simulink model "TurnLightLogic_backup"  (R2023a)
settings: Solver=FixedStepDiscrete  StartTime=0.0  StopTime=10.0  FixedStep=0.01  RelTol=1e-3
undefined symbols (not defined in the file or in its folder): ComplexTurnLightOnOff, ComplexTurnLightPosition, TurnLightCtrlPara, TurnLightService_TurnLightControl_Operation_Operation
settings Model: Creator=19856  LastModifiedBy=19856
settings DataIOCC: SaveFormat=StructureWithTime
settings OptimizationCC: DefaultParameterBehavior=Inlined  EnhancedBackFolding=on  PassReuseOutputArgsAs=Individual arguments  ZeroExternalMemoryAtStartup=off  ZeroInternalMemoryAtStartup=off  OptimizeBlockOrder=speed  DifferentSizesBufferReuse=on  OptimizationCustomize=off  EfficientTunableParamExpr=on
settings DebuggingCC: ParameterTunabilityLossMsg=error
settings ModelReferenceCC: ModelReferenceNumInstancesAllowed=Single
settings SFSimCC: MATLABDynamicMemAlloc=off
settings RTWCC: Description=AUTOSAR  SystemTargetFile=autosar.tlc  GenCodeOnly=on  TemplateMakefile=ert_default_tmf
settings CodeAppCC: ForceParamTrailComments=on  IgnoreCustomStorageClasses=off  OperatorAnnotations=on  SimulinkDataObjDesc=on  SFDataObjDesc=on  InsertBlockDesc=on
settings STFCustomTargetCC: MultiwordLength=256  ParMdlRefBuildCompliant=on  CompOptLevelCompliant=on  ConcurrentExecutionCompliant=off  IncludeMdlTerminateFcn=off  CombineOutputUpdateFcns=on  SuppressErrorStatus=on  ERTCustomFileBanners=on  SupportNonFinite=off  SupportComplex=off  SupportContinuousTime=off  SupportNonInlinedSFcns=off  RemoveResetFunc=on  MATLABClassNameForMDSCustomization=Simulink.SoftwareTarget.ERTCustomization  AutosarCompliant=on  GRTInterface=off  LookupTableObjectStructAxisOrder=2,1,3,4,...  LUTObjectStructOrderEvenSpacing=Size,Table,Breakpoints  SystemTargetFile=autosar.tlc
settings ERTTargetCC: TargetLangStandard=C99 (ISO)  ConcurrentExecutionCompliant=off  IncludeMdlTerminateFcn=off  SuppressErrorStatus=on  SupportNonFinite=off  SupportComplex=off  ModelStepFunctionPrototypeControlCompliant=off  CPPClassGenCompliant=off  AutosarCompliant=on  LookupTableObjectStructAxisOrder=2,1,3,4,...  LUTObjectStructOrderEvenSpacing=Size,Table,Breakpoints  InlinedParameterPlacement=NonHierarchical  ERTCustomFileTemplate=example_file_process.tlc

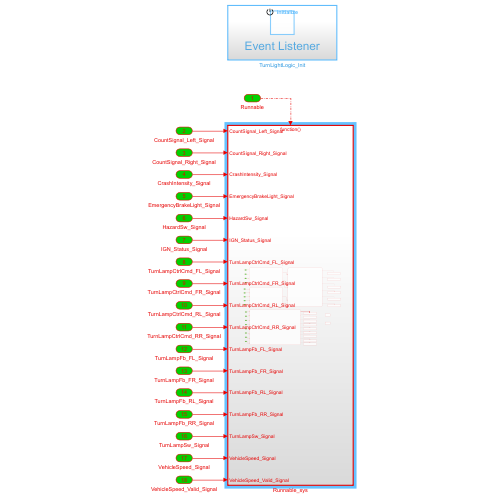
[thumbnail: Simulink's stored preview of the top-level diagram]
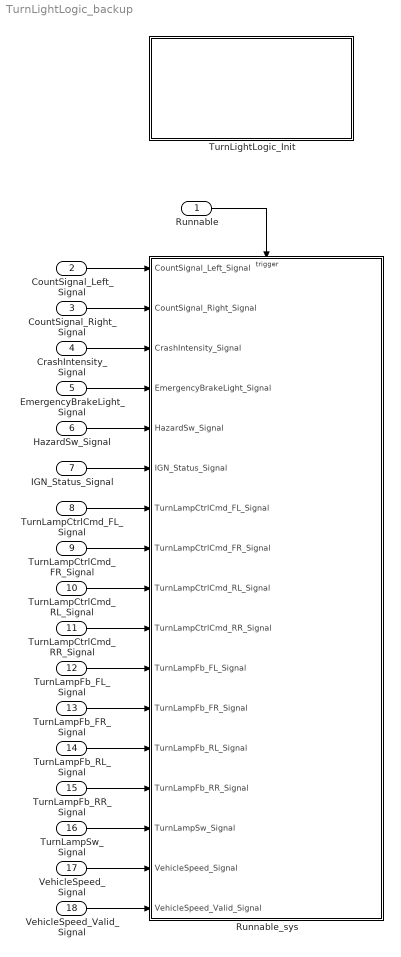
== system TurnLightLogic_backup ==
  Runnable : Inport  SampleTime=0.01  OutputFunctionCall=on
  CountSignal_Left_Signal : Inport  Port=2  OutDataTypeStr=uint8  PortDimensions=1
  CountSignal_Right_Signal : Inport  Port=3  OutDataTypeStr=uint8  PortDimensions=1
  CrashIntensity_Signal : Inport  Port=4  OutDataTypeStr=uint8  PortDimensions=1
  EmergencyBrakeLight_Signal : Inport  Port=5  OutDataTypeStr=uint8  PortDimensions=1
  HazardSw_Signal : Inport  Port=6  OutDataTypeStr=uint8  PortDimensions=1
  IGN_Status_Signal : Inport  Port=7  OutDataTypeStr=uint8  PortDimensions=1
  TurnLampCtrlCmd_FL_Signal : Inport  Port=8  OutDataTypeStr=uint8  PortDimensions=1
  TurnLampCtrlCmd_FR_Signal : Inport  Port=9  OutDataTypeStr=uint8  PortDimensions=1
  TurnLampCtrlCmd_RL_Signal : Inport  Port=10  OutDataTypeStr=uint8  PortDimensions=1
  TurnLampCtrlCmd_RR_Signal : Inport  Port=11  OutDataTypeStr=uint8  PortDimensions=1
  TurnLampFb_FL_Signal : Inport  Port=12  OutDataTypeStr=uint8  PortDimensions=1
  TurnLampFb_FR_Signal : Inport  Port=13  OutDataTypeStr=uint8  PortDimensions=1
  TurnLampFb_RL_Signal : Inport  Port=14  OutDataTypeStr=uint8  PortDimensions=1
  TurnLampFb_RR_Signal : Inport  Port=15  OutDataTypeStr=uint8  PortDimensions=1
  TurnLampSw_Signal : Inport  Port=16  OutDataTypeStr=uint8  PortDimensions=1
  VehicleSpeed_Signal : Inport  Port=17  OutDataTypeStr=uint8  PortDimensions=1
  VehicleSpeed_Valid_Signal : Inport  Port=18  OutDataTypeStr=uint8  PortDimensions=1
  Runnable_sys : Subsystem
  TurnLightLogic_Init : Subsystem
  wires:
  CountSignal_Left_Signal/1 -> Runnable_sys/1(CountSignal_Left_Signal)
  CountSignal_Right_Signal/1 -> Runnable_sys/2(CountSignal_Right_Signal)
  CrashIntensity_Signal/1 -> Runnable_sys/3(CrashIntensity_Signal)
  EmergencyBrakeLight_Signal/1 -> Runnable_sys/4(EmergencyBrakeLight_Signal)
  HazardSw_Signal/1 -> Runnable_sys/5(HazardSw_Signal)
  IGN_Status_Signal/1 -> Runnable_sys/6(IGN_Status_Signal)
  TurnLampCtrlCmd_FL_Signal/1 -> Runnable_sys/7(TurnLampCtrlCmd_FL_Signal)
  TurnLampCtrlCmd_FR_Signal/1 -> Runnable_sys/8(TurnLampCtrlCmd_FR_Signal)
  TurnLampCtrlCmd_RL_Signal/1 -> Runnable_sys/9(TurnLampCtrlCmd_RL_Signal)
  TurnLampCtrlCmd_RR_Signal/1 -> Runnable_sys/10(TurnLampCtrlCmd_RR_Signal)
  TurnLampFb_FL_Signal/1 -> Runnable_sys/11(TurnLampFb_FL_Signal)
  TurnLampFb_FR_Signal/1 -> Runnable_sys/12(TurnLampFb_FR_Signal)
  TurnLampFb_RL_Signal/1 -> Runnable_sys/13(TurnLampFb_RL_Signal)
  TurnLampFb_RR_Signal/1 -> Runnable_sys/14(TurnLampFb_RR_Signal)
  TurnLampSw_Signal/1 -> Runnable_sys/15(TurnLampSw_Signal)
  VehicleSpeed_Signal/1 -> Runnable_sys/16(VehicleSpeed_Signal)
  VehicleSpeed_Valid_Signal/1 -> Runnable_sys/17(VehicleSpeed_Valid_Signal)
  Runnable/1 -> Runnable_sys/Trigger

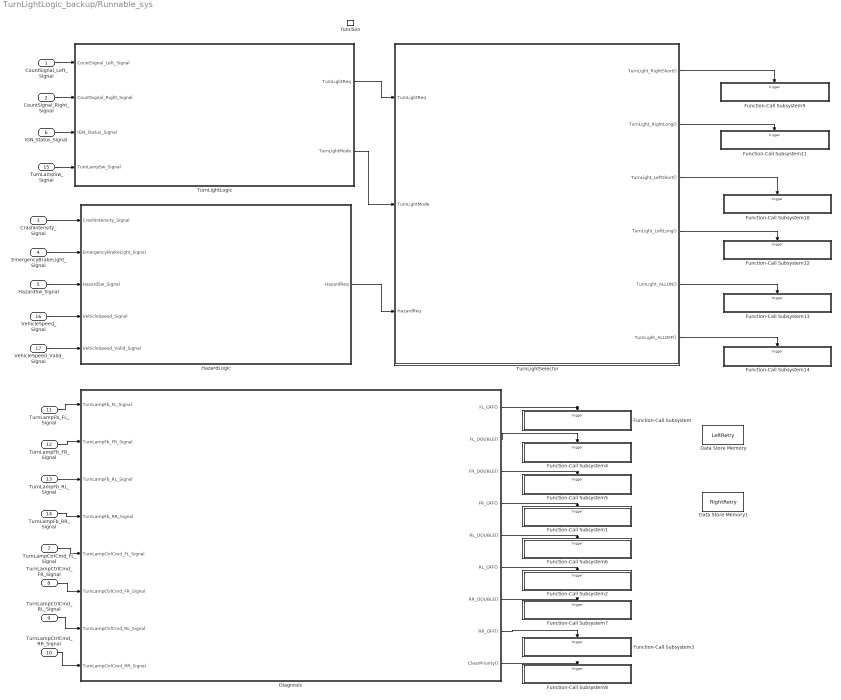
== system TurnLightLogic_backup/Runnable_sys ==
  CountSignal_Left_Signal : Inport
  CountSignal_Right_Signal : Inport  Port=2
  CrashIntensity_Signal : Inport  Port=3
  EmergencyBrakeLight_Signal : Inport  Port=4
  HazardSw_Signal : Inport  Port=5
  IGN_Status_Signal : Inport  Port=6
  TurnLampCtrlCmd_FL_Signal : Inport  Port=7
  TurnLampCtrlCmd_FR_Signal : Inport  Port=8
  TurnLampCtrlCmd_RL_Signal : Inport  Port=9
  TurnLampCtrlCmd_RR_Signal : Inport  Port=10
  TurnLampFb_FL_Signal : Inport  Port=11
  TurnLampFb_FR_Signal : Inport  Port=12
  TurnLampFb_RL_Signal : Inport  Port=13
  TurnLampFb_RR_Signal : Inport  Port=14
  TurnLampSw_Signal : Inport  Port=15
  VehicleSpeed_Signal : Inport  Port=16  OutDataTypeStr=uint8
  VehicleSpeed_Valid_Signal : Inport  Port=17
  function : TriggerPort  TriggerType=function-call  VariantControl=(inherit)  SampleTimeType=periodic  SampleTime=-1
  Data Store Memory : DataStoreMemory  DataStoreName=LeftRetry  WriteAfterWriteMsg=warning  ShowAdditionalParam=off  OutDataTypeStr=uint8
  Data Store Memory1 : DataStoreMemory  DataStoreName=RightRetry  WriteAfterWriteMsg=warning  ShowAdditionalParam=off  OutDataTypeStr=uint8
  Diagnosis : Stateflow chart  TreatAsAtomicUnit=on
  Function-Call Subsystem : Subsystem  TreatAsAtomicUnit=on
  Function-Call Subsystem1 : Subsystem  TreatAsAtomicUnit=on
  Function-Call Subsystem10 : Subsystem  TreatAsAtomicUnit=on
  Function-Call Subsystem11 : Subsystem  TreatAsAtomicUnit=on
  Function-Call Subsystem12 : Subsystem  TreatAsAtomicUnit=on
  Function-Call Subsystem13 : Subsystem  TreatAsAtomicUnit=on
  Function-Call Subsystem14 : Subsystem  TreatAsAtomicUnit=on
  Function-Call Subsystem2 : Subsystem  TreatAsAtomicUnit=on
  Function-Call Subsystem3 : Subsystem  TreatAsAtomicUnit=on
  Function-Call Subsystem4 : Subsystem  TreatAsAtomicUnit=on
  Function-Call Subsystem5 : Subsystem  TreatAsAtomicUnit=on
  Function-Call Subsystem6 : Subsystem  TreatAsAtomicUnit=on
  Function-Call Subsystem7 : Subsystem  TreatAsAtomicUnit=on
  Function-Call Subsystem8 : Subsystem  TreatAsAtomicUnit=on
  Function-Call Subsystem9 : Subsystem  TreatAsAtomicUnit=on
  HazardLogic : Stateflow chart  TreatAsAtomicUnit=on
  TurnLightLogic : Stateflow chart  TreatAsAtomicUnit=on
  TurnLightSelector : Stateflow chart  TreatAsAtomicUnit=on
  wires:
  CountSignal_Left_Signal/1 -> TurnLightLogic/1(CountSignal_Left_Signal)
  CountSignal_Right_Signal/1 -> TurnLightLogic/2(CountSignal_Right_Signal)
  CrashIntensity_Signal/1 -> HazardLogic/1(CrashIntensity_Signal)
  EmergencyBrakeLight_Signal/1 -> HazardLogic/2(EmergencyBrakeLight_Signal)
  HazardSw_Signal/1 -> HazardLogic/3(HazardSw_Signal)
  IGN_Status_Signal/1 -> TurnLightLogic/3(IGN_Status_Signal)
  TurnLampFb_FL_Signal/1 -> Diagnosis/1(TurnLampFb_FL_Signal)
  TurnLampFb_FR_Signal/1 -> Diagnosis/2(TurnLampFb_FR_Signal)
  TurnLampFb_RL_Signal/1 -> Diagnosis/3(TurnLampFb_RL_Signal)
  TurnLampFb_RR_Signal/1 -> Diagnosis/4(TurnLampFb_RR_Signal)
  TurnLampSw_Signal/1 -> TurnLightLogic/4(TurnLampSw_Signal)
  VehicleSpeed_Signal/1 -> HazardLogic/4(VehicleSpeed_Signal)
  VehicleSpeed_Valid_Signal/1 -> HazardLogic/5(VehicleSpeed_Valid_Signal)
  TurnLightLogic/1(TurnLightReq) -> TurnLightSelector/1(TurnLightReq)
  TurnLightLogic/2(TurnLightMode) -> TurnLightSelector/2(TurnLightMode)
  HazardLogic/1(HazardReq) -> TurnLightSelector/3(HazardReq)
  TurnLampCtrlCmd_FL_Signal/1 -> Diagnosis/5(TurnLampCtrlCmd_FL_Signal)
  TurnLampCtrlCmd_FR_Signal/1 -> Diagnosis/6(TurnLampCtrlCmd_FR_Signal)
  TurnLampCtrlCmd_RL_Signal/1 -> Diagnosis/7(TurnLampCtrlCmd_RL_Signal)
  TurnLampCtrlCmd_RR_Signal/1 -> Diagnosis/8(TurnLampCtrlCmd_RR_Signal)
  TurnLightSelector/6(TurnLight_ALLOFF()) -> Function-Call Subsystem14/Trigger
  TurnLightSelector/5(TurnLight_ALLON()) -> Function-Call Subsystem13/Trigger
  TurnLightSelector/4(TurnLight_LeftLong()) -> Function-Call Subsystem12/Trigger
  TurnLightSelector/3(TurnLight_LeftShort()) -> Function-Call Subsystem10/Trigger
  TurnLightSelector/2(TurnLight_RightLong()) -> Function-Call Subsystem11/Trigger
  TurnLightSelector/1(TurnLight_RightShort()) -> Function-Call Subsystem9/Trigger
  Diagnosis/1(FL_OFF()) -> Function-Call Subsystem/Trigger
  Diagnosis/2(FL_DOUBLE()) -> Function-Call Subsystem4/Trigger
  Diagnosis/3(FR_DOUBLE()) -> Function-Call Subsystem5/Trigger
  Diagnosis/4(FR_OFF()) -> Function-Call Subsystem1/Trigger
  Diagnosis/5(RL_DOUBLE()) -> Function-Call Subsystem6/Trigger
  Diagnosis/6(RL_OFF()) -> Function-Call Subsystem2/Trigger
  Diagnosis/7(RR_DOUBLE()) -> Function-Call Subsystem7/Trigger
  Diagnosis/8(RR_OFF()) -> Function-Call Subsystem3/Trigger
  Diagnosis/9(ClearPriority()) -> Function-Call Subsystem8/Trigger

== system TurnLightLogic_backup/TurnLightLogic_Init ==
  Event Listener : EventListener  EventName=reset

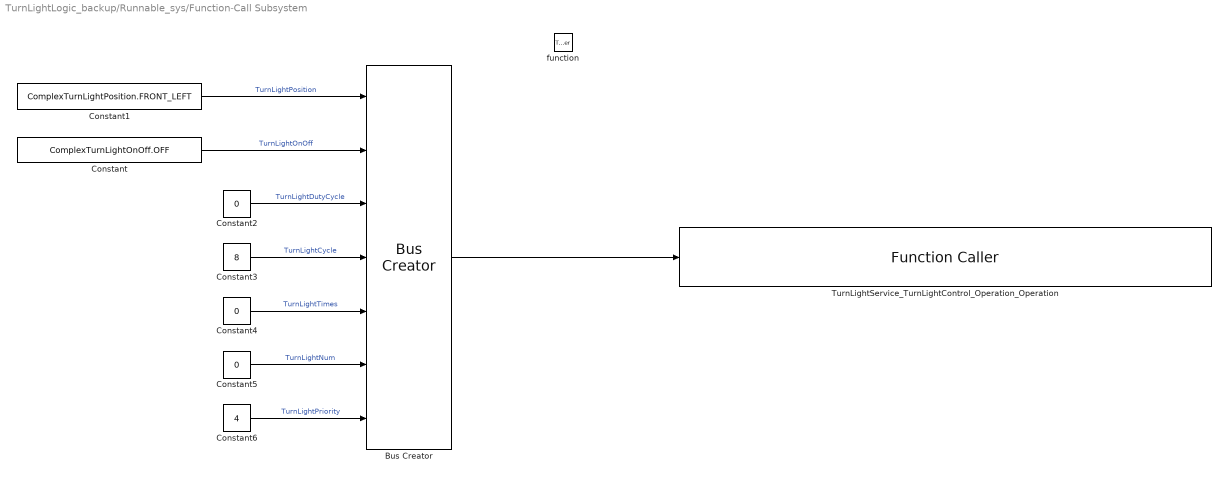
== system TurnLightLogic_backup/Runnable_sys/Function-Call Subsystem ==
  function : TriggerPort  TriggerType=function-call  VariantControl=(inherit)
  Bus Creator : BusCreator  Inputs=7  OutDataTypeStr=Bus: TurnLightService  NonVirtualBus=on
  Constant : Constant  Value=ComplexTurnLightOnOff.OFF  OutDataTypeStr=Enum: ComplexTurnLightOnOff
  Constant1 : Constant  Value=ComplexTurnLightPosition.FRONT_LEFT  OutDataTypeStr=Enum:ComplexTurnLightPosition
  Constant2 : Constant  Value=0  OutDataTypeStr=uint8
  Constant3 : Constant  Value=8  OutDataTypeStr=uint8
  Constant4 : Constant  Value=0  OutDataTypeStr=uint8
  Constant5 : Constant  Value=0  OutDataTypeStr=uint8
  Constant6 : Constant  Value=4  VectorParams1D=off  OutDataTypeStr=uint8
  TurnLightService_TurnLightControl_Operation_Operation : FunctionCaller  FunctionPrototype=TurnLightService_TurnLightControl_Operation_Operation(TurnLightCtrlPara)  InputArgumentSpecifications=P_TurnLightService_Ctrl_Oeration
  wires:
  Constant5/1 -> Bus Creator/6  "TurnLightNum"
  Bus Creator/1 -> TurnLightService_TurnLightControl_Operation_Operation/1
  Constant/1 -> Bus Creator/2  "TurnLightOnOff"
  Constant1/1 -> Bus Creator/1  "TurnLightPosition"
  Constant3/1 -> Bus Creator/4  "TurnLightCycle"
  Constant4/1 -> Bus Creator/5  "TurnLightTimes"
  Constant2/1 -> Bus Creator/3  "TurnLightDutyCycle"
  Constant6/1 -> Bus Creator/7  "TurnLightPriority"

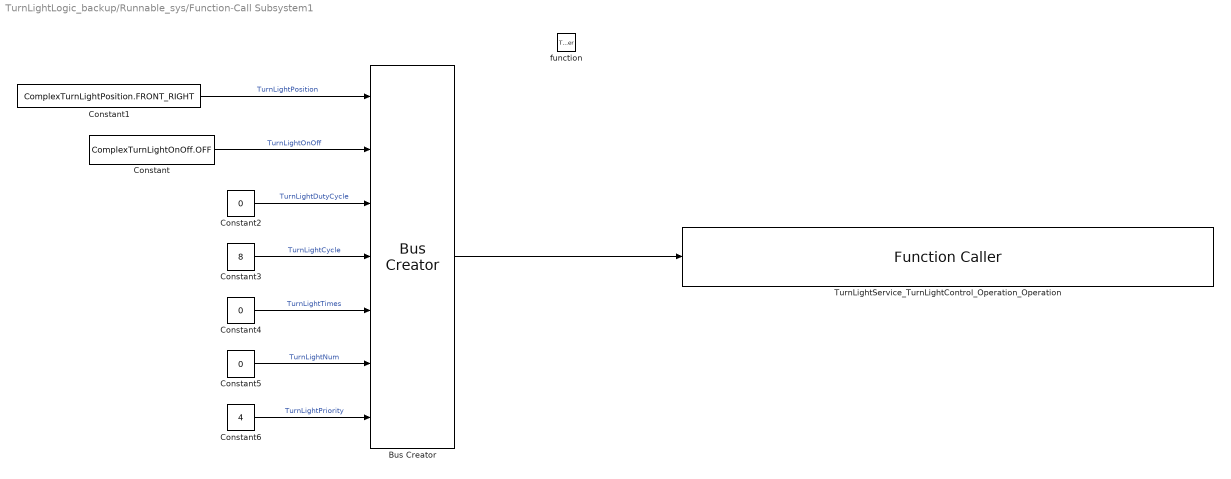
== system TurnLightLogic_backup/Runnable_sys/Function-Call Subsystem1 ==
  function : TriggerPort  TriggerType=function-call  VariantControl=(inherit)
  Bus Creator : BusCreator  Inputs=7  OutDataTypeStr=Bus: TurnLightService  NonVirtualBus=on
  Constant : Constant  Value=ComplexTurnLightOnOff.OFF  OutDataTypeStr=Enum: ComplexTurnLightOnOff
  Constant1 : Constant  Value=ComplexTurnLightPosition.FRONT_RIGHT  OutDataTypeStr=Enum:ComplexTurnLightPosition
  Constant2 : Constant  Value=0  OutDataTypeStr=uint8
  Constant3 : Constant  Value=8  OutDataTypeStr=uint8
  Constant4 : Constant  Value=0  OutDataTypeStr=uint8
  Constant5 : Constant  Value=0  OutDataTypeStr=uint8
  Constant6 : Constant  Value=4  VectorParams1D=off  OutDataTypeStr=uint8
  TurnLightService_TurnLightControl_Operation_Operation : FunctionCaller  FunctionPrototype=TurnLightService_TurnLightControl_Operation_Operation(TurnLightCtrlPara)  InputArgumentSpecifications=P_TurnLightService_Ctrl_Oeration
  wires:
  Constant6/1 -> Bus Creator/7  "TurnLightPriority"
  Constant2/1 -> Bus Creator/3  "TurnLightDutyCycle"
  Constant4/1 -> Bus Creator/5  "TurnLightTimes"
  Constant3/1 -> Bus Creator/4  "TurnLightCycle"
  Constant1/1 -> Bus Creator/1  "TurnLightPosition"
  Constant/1 -> Bus Creator/2  "TurnLightOnOff"
  Bus Creator/1 -> TurnLightService_TurnLightControl_Operation_Operation/1
  Constant5/1 -> Bus Creator/6  "TurnLightNum"

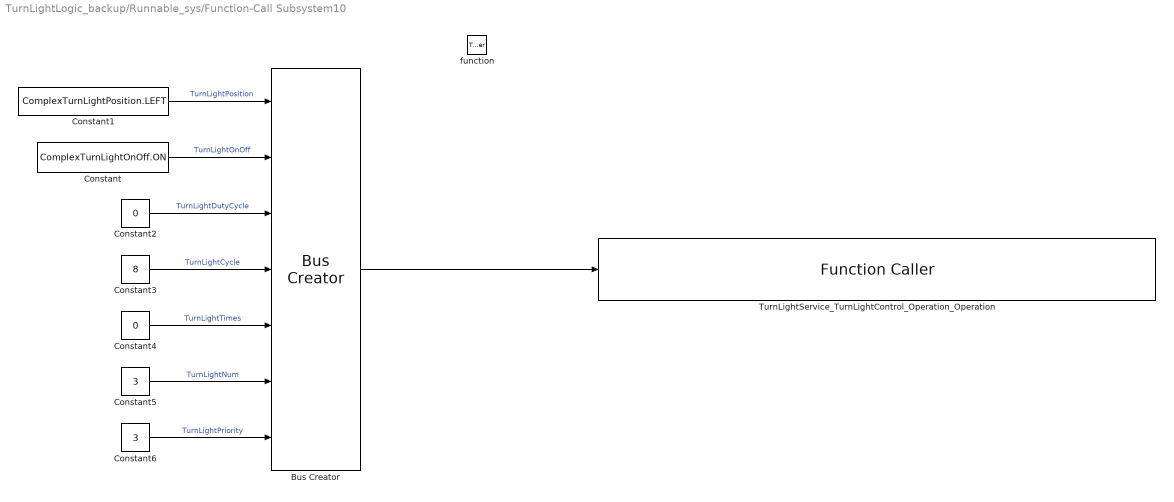
== system TurnLightLogic_backup/Runnable_sys/Function-Call Subsystem10 ==
  function : TriggerPort  TriggerType=function-call  VariantControl=(inherit)
  Bus Creator : BusCreator  Inputs=7  OutDataTypeStr=Bus: TurnLightService  NonVirtualBus=on
  Constant : Constant  Value=ComplexTurnLightOnOff.ON  OutDataTypeStr=Enum: ComplexTurnLightOnOff
  Constant1 : Constant  Value=ComplexTurnLightPosition.LEFT  OutDataTypeStr=Enum:ComplexTurnLightPosition
  Constant2 : Constant  Value=0  OutDataTypeStr=uint8
  Constant3 : Constant  Value=8  OutDataTypeStr=uint8
  Constant4 : Constant  Value=0  OutDataTypeStr=uint8
  Constant5 : Constant  Value=3  OutDataTypeStr=uint8
  Constant6 : Constant  Value=3  VectorParams1D=off  OutDataTypeStr=uint8
  TurnLightService_TurnLightControl_Operation_Operation : FunctionCaller  FunctionPrototype=TurnLightService_TurnLightControl_Operation_Operation(TurnLightCtrlPara)  InputArgumentSpecifications=P_TurnLightService_Ctrl_Oeration
  wires:
  Constant5/1 -> Bus Creator/6  "TurnLightNum"
  Bus Creator/1 -> TurnLightService_TurnLightControl_Operation_Operation/1
  Constant/1 -> Bus Creator/2  "TurnLightOnOff"
  Constant1/1 -> Bus Creator/1  "TurnLightPosition"
  Constant3/1 -> Bus Creator/4  "TurnLightCycle"
  Constant4/1 -> Bus Creator/5  "TurnLightTimes"
  Constant2/1 -> Bus Creator/3  "TurnLightDutyCycle"
  Constant6/1 -> Bus Creator/7  "TurnLightPriority"

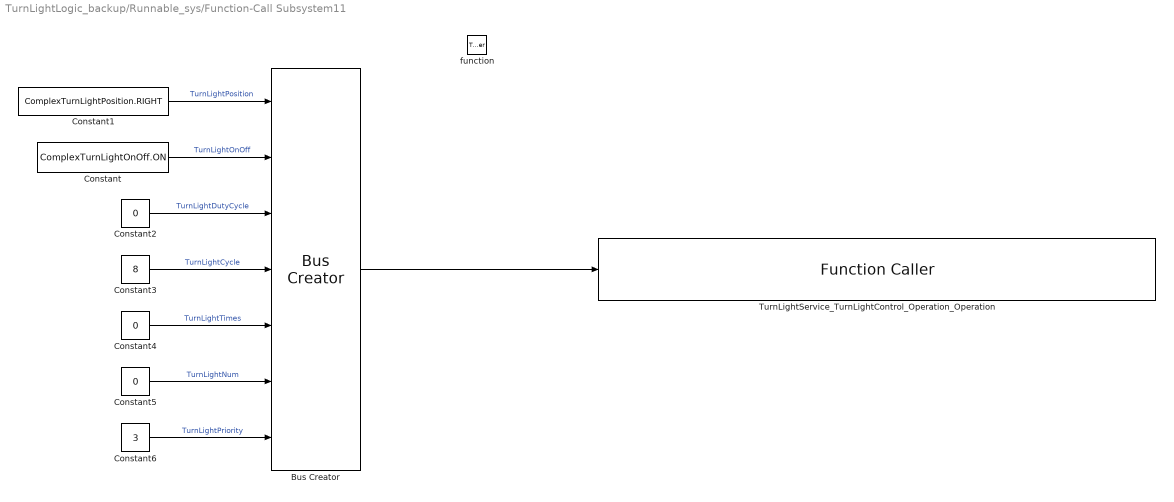
== system TurnLightLogic_backup/Runnable_sys/Function-Call Subsystem11 ==
  function : TriggerPort  TriggerType=function-call  VariantControl=(inherit)
  Bus Creator : BusCreator  Inputs=7  OutDataTypeStr=Bus: TurnLightService  NonVirtualBus=on
  Constant : Constant  Value=ComplexTurnLightOnOff.ON  OutDataTypeStr=Enum: ComplexTurnLightOnOff
  Constant1 : Constant  Value=ComplexTurnLightPosition.RIGHT  OutDataTypeStr=Enum:ComplexTurnLightPosition
  Constant2 : Constant  Value=0  OutDataTypeStr=uint8
  Constant3 : Constant  Value=8  OutDataTypeStr=uint8
  Constant4 : Constant  Value=0  OutDataTypeStr=uint8
  Constant5 : Constant  Value=0  OutDataTypeStr=uint8
  Constant6 : Constant  Value=3  VectorParams1D=off  OutDataTypeStr=uint8
  TurnLightService_TurnLightControl_Operation_Operation : FunctionCaller  FunctionPrototype=TurnLightService_TurnLightControl_Operation_Operation(TurnLightCtrlPara)  InputArgumentSpecifications=P_TurnLightService_Ctrl_Oeration
  wires:
  Constant5/1 -> Bus Creator/6  "TurnLightNum"
  Bus Creator/1 -> TurnLightService_TurnLightControl_Operation_Operation/1
  Constant/1 -> Bus Creator/2  "TurnLightOnOff"
  Constant1/1 -> Bus Creator/1  "TurnLightPosition"
  Constant3/1 -> Bus Creator/4  "TurnLightCycle"
  Constant4/1 -> Bus Creator/5  "TurnLightTimes"
  Constant2/1 -> Bus Creator/3  "TurnLightDutyCycle"
  Constant6/1 -> Bus Creator/7  "TurnLightPriority"

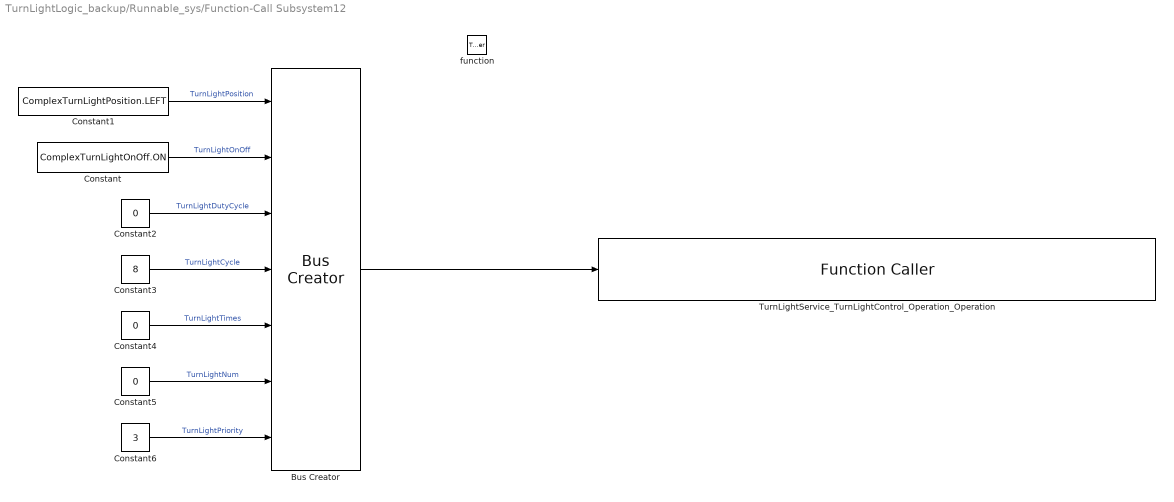
== system TurnLightLogic_backup/Runnable_sys/Function-Call Subsystem12 ==
  function : TriggerPort  TriggerType=function-call  VariantControl=(inherit)
  Bus Creator : BusCreator  Inputs=7  OutDataTypeStr=Bus: TurnLightService  NonVirtualBus=on
  Constant : Constant  Value=ComplexTurnLightOnOff.ON  OutDataTypeStr=Enum: ComplexTurnLightOnOff
  Constant1 : Constant  Value=ComplexTurnLightPosition.LEFT  OutDataTypeStr=Enum:ComplexTurnLightPosition
  Constant2 : Constant  Value=0  OutDataTypeStr=uint8
  Constant3 : Constant  Value=8  OutDataTypeStr=uint8
  Constant4 : Constant  Value=0  OutDataTypeStr=uint8
  Constant5 : Constant  Value=0  OutDataTypeStr=uint8
  Constant6 : Constant  Value=3  VectorParams1D=off  OutDataTypeStr=uint8
  TurnLightService_TurnLightControl_Operation_Operation : FunctionCaller  FunctionPrototype=TurnLightService_TurnLightControl_Operation_Operation(TurnLightCtrlPara)  InputArgumentSpecifications=P_TurnLightService_Ctrl_Oeration
  wires:
  Constant6/1 -> Bus Creator/7  "TurnLightPriority"
  Constant2/1 -> Bus Creator/3  "TurnLightDutyCycle"
  Constant4/1 -> Bus Creator/5  "TurnLightTimes"
  Constant3/1 -> Bus Creator/4  "TurnLightCycle"
  Constant1/1 -> Bus Creator/1  "TurnLightPosition"
  Constant/1 -> Bus Creator/2  "TurnLightOnOff"
  Bus Creator/1 -> TurnLightService_TurnLightControl_Operation_Operation/1
  Constant5/1 -> Bus Creator/6  "TurnLightNum"

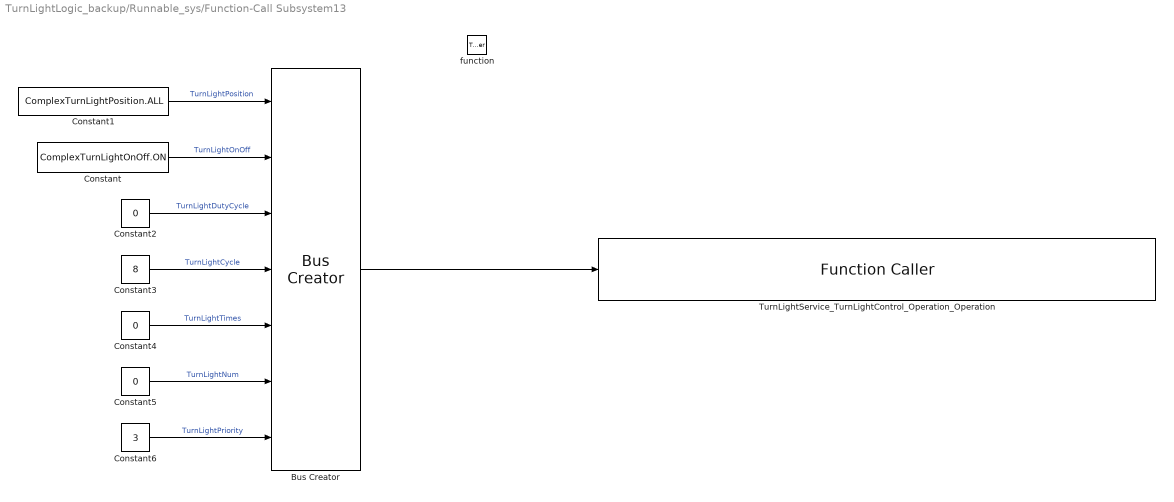
== system TurnLightLogic_backup/Runnable_sys/Function-Call Subsystem13 ==
  function : TriggerPort  TriggerType=function-call  VariantControl=(inherit)
  Bus Creator : BusCreator  Inputs=7  OutDataTypeStr=Bus: TurnLightService  NonVirtualBus=on
  Constant : Constant  Value=ComplexTurnLightOnOff.ON  OutDataTypeStr=Enum: ComplexTurnLightOnOff
  Constant1 : Constant  Value=ComplexTurnLightPosition.ALL  OutDataTypeStr=Enum:ComplexTurnLightPosition
  Constant2 : Constant  Value=0  OutDataTypeStr=uint8
  Constant3 : Constant  Value=8  OutDataTypeStr=uint8
  Constant4 : Constant  Value=0  OutDataTypeStr=uint8
  Constant5 : Constant  Value=0  OutDataTypeStr=uint8
  Constant6 : Constant  Value=3  VectorParams1D=off  OutDataTypeStr=uint8
  TurnLightService_TurnLightControl_Operation_Operation : FunctionCaller  FunctionPrototype=TurnLightService_TurnLightControl_Operation_Operation(TurnLightCtrlPara)  InputArgumentSpecifications=P_TurnLightService_Ctrl_Oeration
  wires:
  Constant5/1 -> Bus Creator/6  "TurnLightNum"
  Bus Creator/1 -> TurnLightService_TurnLightControl_Operation_Operation/1
  Constant/1 -> Bus Creator/2  "TurnLightOnOff"
  Constant1/1 -> Bus Creator/1  "TurnLightPosition"
  Constant3/1 -> Bus Creator/4  "TurnLightCycle"
  Constant4/1 -> Bus Creator/5  "TurnLightTimes"
  Constant2/1 -> Bus Creator/3  "TurnLightDutyCycle"
  Constant6/1 -> Bus Creator/7  "TurnLightPriority"

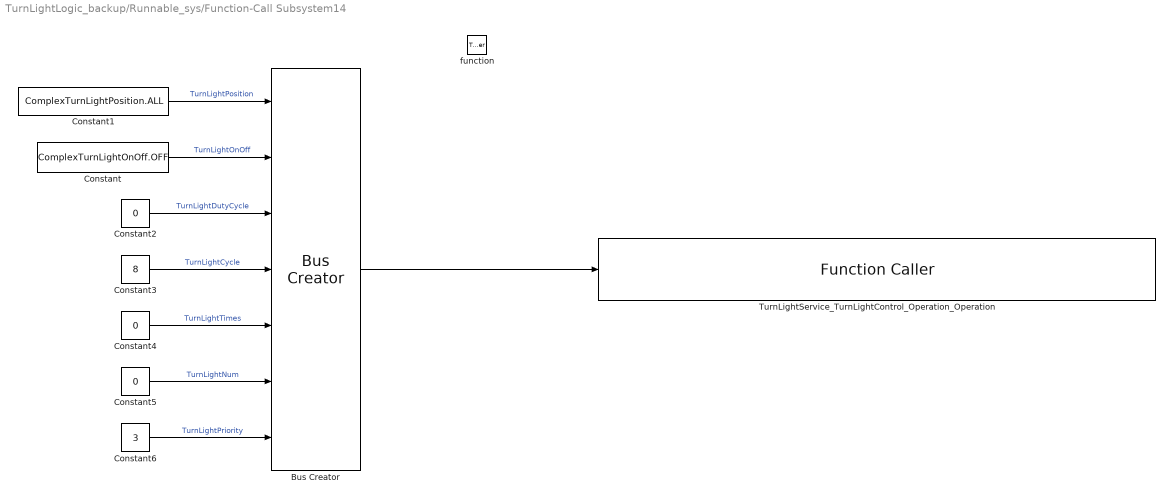
== system TurnLightLogic_backup/Runnable_sys/Function-Call Subsystem14 ==
  function : TriggerPort  TriggerType=function-call  VariantControl=(inherit)
  Bus Creator : BusCreator  Inputs=7  OutDataTypeStr=Bus: TurnLightService  NonVirtualBus=on
  Constant : Constant  Value=ComplexTurnLightOnOff.OFF  OutDataTypeStr=Enum: ComplexTurnLightOnOff
  Constant1 : Constant  Value=ComplexTurnLightPosition.ALL  OutDataTypeStr=Enum:ComplexTurnLightPosition
  Constant2 : Constant  Value=0  OutDataTypeStr=uint8
  Constant3 : Constant  Value=8  OutDataTypeStr=uint8
  Constant4 : Constant  Value=0  OutDataTypeStr=uint8
  Constant5 : Constant  Value=0  OutDataTypeStr=uint8
  Constant6 : Constant  Value=3  VectorParams1D=off  OutDataTypeStr=uint8
  TurnLightService_TurnLightControl_Operation_Operation : FunctionCaller  FunctionPrototype=TurnLightService_TurnLightControl_Operation_Operation(TurnLightCtrlPara)  InputArgumentSpecifications=P_TurnLightService_Ctrl_Oeration
  wires:
  Constant6/1 -> Bus Creator/7  "TurnLightPriority"
  Constant2/1 -> Bus Creator/3  "TurnLightDutyCycle"
  Constant4/1 -> Bus Creator/5  "TurnLightTimes"
  Constant3/1 -> Bus Creator/4  "TurnLightCycle"
  Constant1/1 -> Bus Creator/1  "TurnLightPosition"
  Constant/1 -> Bus Creator/2  "TurnLightOnOff"
  Bus Creator/1 -> TurnLightService_TurnLightControl_Operation_Operation/1
  Constant5/1 -> Bus Creator/6  "TurnLightNum"

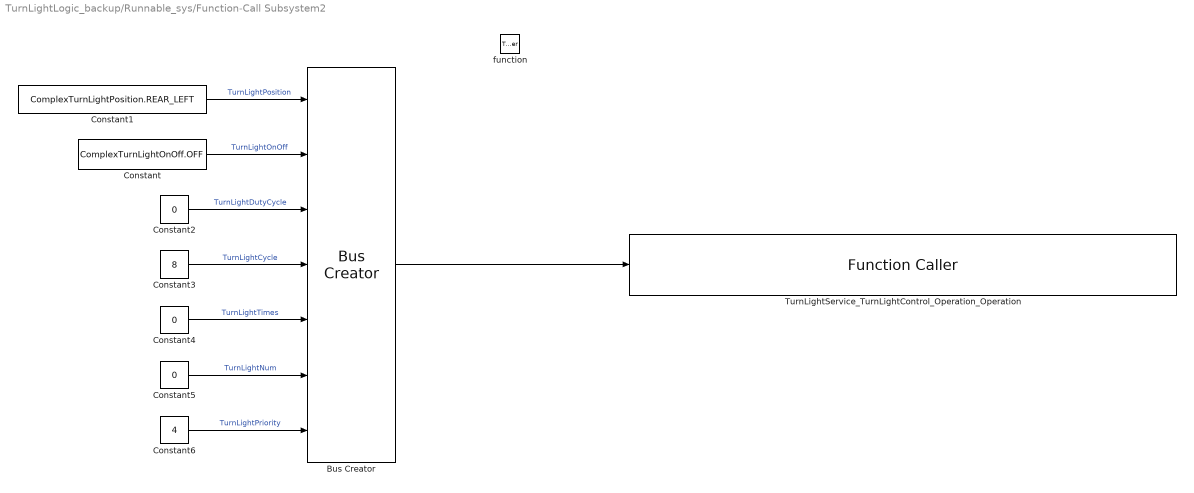
== system TurnLightLogic_backup/Runnable_sys/Function-Call Subsystem2 ==
  function : TriggerPort  TriggerType=function-call  VariantControl=(inherit)
  Bus Creator : BusCreator  Inputs=7  OutDataTypeStr=Bus: TurnLightService  NonVirtualBus=on
  Constant : Constant  Value=ComplexTurnLightOnOff.OFF  OutDataTypeStr=Enum: ComplexTurnLightOnOff
  Constant1 : Constant  Value=ComplexTurnLightPosition.REAR_LEFT  OutDataTypeStr=Enum:ComplexTurnLightPosition
  Constant2 : Constant  Value=0  OutDataTypeStr=uint8
  Constant3 : Constant  Value=8  OutDataTypeStr=uint8
  Constant4 : Constant  Value=0  OutDataTypeStr=uint8
  Constant5 : Constant  Value=0  OutDataTypeStr=uint8
  Constant6 : Constant  Value=4  VectorParams1D=off  OutDataTypeStr=uint8
  TurnLightService_TurnLightControl_Operation_Operation : FunctionCaller  FunctionPrototype=TurnLightService_TurnLightControl_Operation_Operation(TurnLightCtrlPara)  InputArgumentSpecifications=P_TurnLightService_Ctrl_Oeration
  wires:
  Constant5/1 -> Bus Creator/6  "TurnLightNum"
  Bus Creator/1 -> TurnLightService_TurnLightControl_Operation_Operation/1
  Constant/1 -> Bus Creator/2  "TurnLightOnOff"
  Constant1/1 -> Bus Creator/1  "TurnLightPosition"
  Constant3/1 -> Bus Creator/4  "TurnLightCycle"
  Constant4/1 -> Bus Creator/5  "TurnLightTimes"
  Constant2/1 -> Bus Creator/3  "TurnLightDutyCycle"
  Constant6/1 -> Bus Creator/7  "TurnLightPriority"

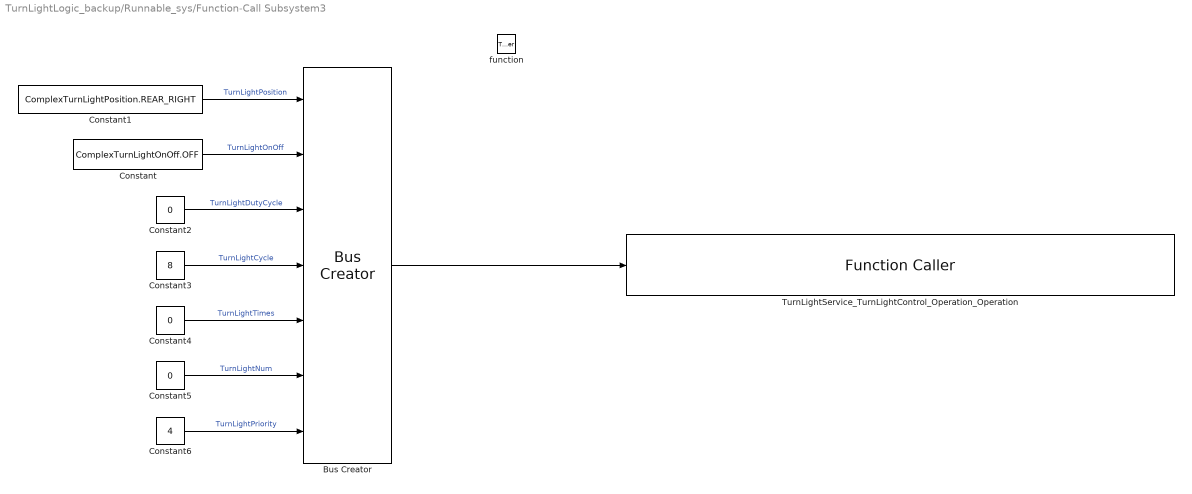
== system TurnLightLogic_backup/Runnable_sys/Function-Call Subsystem3 ==
  function : TriggerPort  TriggerType=function-call  VariantControl=(inherit)
  Bus Creator : BusCreator  Inputs=7  OutDataTypeStr=Bus: TurnLightService  NonVirtualBus=on
  Constant : Constant  Value=ComplexTurnLightOnOff.OFF  OutDataTypeStr=Enum: ComplexTurnLightOnOff
  Constant1 : Constant  Value=ComplexTurnLightPosition.REAR_RIGHT  OutDataTypeStr=Enum:ComplexTurnLightPosition
  Constant2 : Constant  Value=0  OutDataTypeStr=uint8
  Constant3 : Constant  Value=8  OutDataTypeStr=uint8
  Constant4 : Constant  Value=0  OutDataTypeStr=uint8
  Constant5 : Constant  Value=0  OutDataTypeStr=uint8
  Constant6 : Constant  Value=4  VectorParams1D=off  OutDataTypeStr=uint8
  TurnLightService_TurnLightControl_Operation_Operation : FunctionCaller  FunctionPrototype=TurnLightService_TurnLightControl_Operation_Operation(TurnLightCtrlPara)  InputArgumentSpecifications=P_TurnLightService_Ctrl_Oeration
  wires:
  Constant6/1 -> Bus Creator/7  "TurnLightPriority"
  Constant2/1 -> Bus Creator/3  "TurnLightDutyCycle"
  Constant4/1 -> Bus Creator/5  "TurnLightTimes"
  Constant3/1 -> Bus Creator/4  "TurnLightCycle"
  Constant1/1 -> Bus Creator/1  "TurnLightPosition"
  Constant/1 -> Bus Creator/2  "TurnLightOnOff"
  Bus Creator/1 -> TurnLightService_TurnLightControl_Operation_Operation/1
  Constant5/1 -> Bus Creator/6  "TurnLightNum"

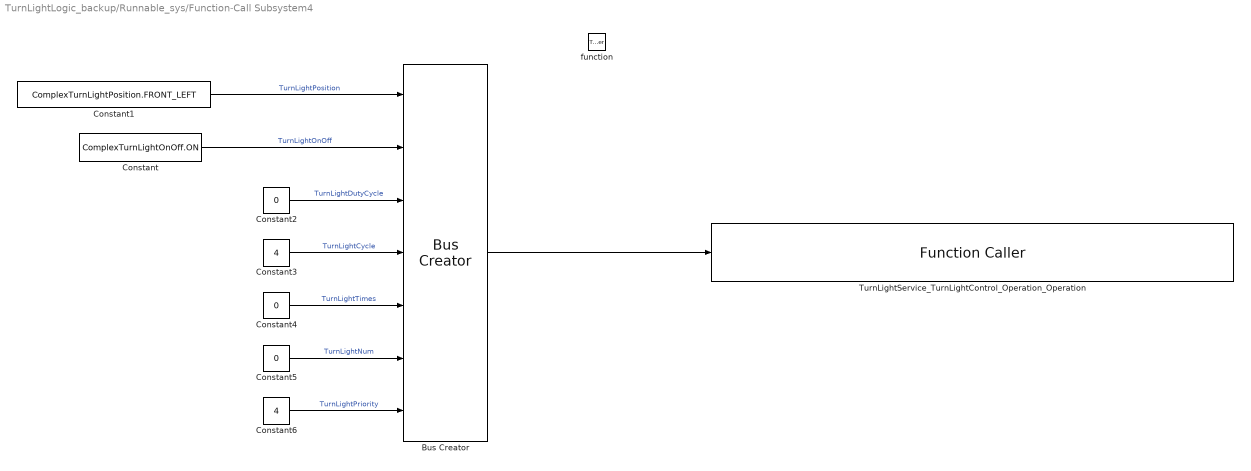
== system TurnLightLogic_backup/Runnable_sys/Function-Call Subsystem4 ==
  function : TriggerPort  TriggerType=function-call  VariantControl=(inherit)
  Bus Creator : BusCreator  Inputs=7  OutDataTypeStr=Bus: TurnLightService  NonVirtualBus=on
  Constant : Constant  Value=ComplexTurnLightOnOff.ON  OutDataTypeStr=Enum: ComplexTurnLightOnOff
  Constant1 : Constant  Value=ComplexTurnLightPosition.FRONT_LEFT  OutDataTypeStr=Enum:ComplexTurnLightPosition
  Constant2 : Constant  Value=0  OutDataTypeStr=uint8
  Constant3 : Constant  Value=4  OutDataTypeStr=uint8
  Constant4 : Constant  Value=0  OutDataTypeStr=uint8
  Constant5 : Constant  Value=0  OutDataTypeStr=uint8
  Constant6 : Constant  Value=4  VectorParams1D=off  OutDataTypeStr=uint8
  TurnLightService_TurnLightControl_Operation_Operation : FunctionCaller  FunctionPrototype=TurnLightService_TurnLightControl_Operation_Operation(TurnLightCtrlPara)  InputArgumentSpecifications=P_TurnLightService_Ctrl_Oeration
  wires:
  Constant6/1 -> Bus Creator/7  "TurnLightPriority"
  Constant2/1 -> Bus Creator/3  "TurnLightDutyCycle"
  Constant4/1 -> Bus Creator/5  "TurnLightTimes"
  Constant3/1 -> Bus Creator/4  "TurnLightCycle"
  Constant1/1 -> Bus Creator/1  "TurnLightPosition"
  Constant/1 -> Bus Creator/2  "TurnLightOnOff"
  Bus Creator/1 -> TurnLightService_TurnLightControl_Operation_Operation/1
  Constant5/1 -> Bus Creator/6  "TurnLightNum"

== system TurnLightLogic_backup/Runnable_sys/Function-Call Subsystem5 ==
  function : TriggerPort  TriggerType=function-call  VariantControl=(inherit)
  Bus Creator : BusCreator  Inputs=7  OutDataTypeStr=Bus: TurnLightService  NonVirtualBus=on
  Constant : Constant  Value=ComplexTurnLightOnOff.ON  OutDataTypeStr=Enum: ComplexTurnLightOnOff
  Constant1 : Constant  Value=ComplexTurnLightPosition.FRONT_RIGHT  OutDataTypeStr=Enum:ComplexTurnLightPosition
  Constant2 : Constant  Value=0  OutDataTypeStr=uint8
  Constant3 : Constant  Value=4  OutDataTypeStr=uint8
  Constant4 : Constant  Value=0  OutDataTypeStr=uint8
  Constant5 : Constant  Value=0  OutDataTypeStr=uint8
  Constant6 : Constant  Value=4  VectorParams1D=off  OutDataTypeStr=uint8
  TurnLightService_TurnLightControl_Operation_Operation : FunctionCaller  FunctionPrototype=TurnLightService_TurnLightControl_Operation_Operation(TurnLightCtrlPara)  InputArgumentSpecifications=P_TurnLightService_Ctrl_Oeration
  wires:
  Constant5/1 -> Bus Creator/6  "TurnLightNum"
  Bus Creator/1 -> TurnLightService_TurnLightControl_Operation_Operation/1
  Constant/1 -> Bus Creator/2  "TurnLightOnOff"
  Constant1/1 -> Bus Creator/1  "TurnLightPosition"
  Constant3/1 -> Bus Creator/4  "TurnLightCycle"
  Constant4/1 -> Bus Creator/5  "TurnLightTimes"
  Constant2/1 -> Bus Creator/3  "TurnLightDutyCycle"
  Constant6/1 -> Bus Creator/7  "TurnLightPriority"

== system TurnLightLogic_backup/Runnable_sys/Function-Call Subsystem6 ==
  function : TriggerPort  TriggerType=function-call  VariantControl=(inherit)
  Bus Creator : BusCreator  Inputs=7  OutDataTypeStr=Bus: TurnLightService  NonVirtualBus=on
  Constant : Constant  Value=ComplexTurnLightOnOff.ON  OutDataTypeStr=Enum: ComplexTurnLightOnOff
  Constant1 : Constant  Value=ComplexTurnLightPosition.REAR_LEFT  OutDataTypeStr=Enum:ComplexTurnLightPosition
  Constant2 : Constant  Value=0  OutDataTypeStr=uint8
  Constant3 : Constant  Value=4  OutDataTypeStr=uint8
  Constant4 : Constant  Value=0  OutDataTypeStr=uint8
  Constant5 : Constant  Value=0  OutDataTypeStr=uint8
  Constant6 : Constant  Value=4  VectorParams1D=off  OutDataTypeStr=uint8
  TurnLightService_TurnLightControl_Operation_Operation : FunctionCaller  FunctionPrototype=TurnLightService_TurnLightControl_Operation_Operation(TurnLightCtrlPara)  InputArgumentSpecifications=P_TurnLightService_Ctrl_Oeration
  wires:
  Constant6/1 -> Bus Creator/7  "TurnLightPriority"
  Constant2/1 -> Bus Creator/3  "TurnLightDutyCycle"
  Constant4/1 -> Bus Creator/5  "TurnLightTimes"
  Constant3/1 -> Bus Creator/4  "TurnLightCycle"
  Constant1/1 -> Bus Creator/1  "TurnLightPosition"
  Constant/1 -> Bus Creator/2  "TurnLightOnOff"
  Bus Creator/1 -> TurnLightService_TurnLightControl_Operation_Operation/1
  Constant5/1 -> Bus Creator/6  "TurnLightNum"

== system TurnLightLogic_backup/Runnable_sys/Function-Call Subsystem7 ==
  function : TriggerPort  TriggerType=function-call  VariantControl=(inherit)
  Bus Creator : BusCreator  Inputs=7  OutDataTypeStr=Bus: TurnLightService  NonVirtualBus=on
  Constant : Constant  Value=ComplexTurnLightOnOff.ON  OutDataTypeStr=Enum: ComplexTurnLightOnOff
  Constant1 : Constant  Value=ComplexTurnLightPosition.REAR_RIGHT  OutDataTypeStr=Enum:ComplexTurnLightPosition
  Constant2 : Constant  Value=0  OutDataTypeStr=uint8
  Constant3 : Constant  Value=4  OutDataTypeStr=uint8
  Constant4 : Constant  Value=0  OutDataTypeStr=uint8
  Constant5 : Constant  Value=0  OutDataTypeStr=uint8
  Constant6 : Constant  Value=4  VectorParams1D=off  OutDataTypeStr=uint8
  TurnLightService_TurnLightControl_Operation_Operation : FunctionCaller  FunctionPrototype=TurnLightService_TurnLightControl_Operation_Operation(TurnLightCtrlPara)  InputArgumentSpecifications=P_TurnLightService_Ctrl_Oeration
  wires:
  Constant5/1 -> Bus Creator/6  "TurnLightNum"
  Bus Creator/1 -> TurnLightService_TurnLightControl_Operation_Operation/1
  Constant/1 -> Bus Creator/2  "TurnLightOnOff"
  Constant1/1 -> Bus Creator/1  "TurnLightPosition"
  Constant3/1 -> Bus Creator/4  "TurnLightCycle"
  Constant4/1 -> Bus Creator/5  "TurnLightTimes"
  Constant2/1 -> Bus Creator/3  "TurnLightDutyCycle"
  Constant6/1 -> Bus Creator/7  "TurnLightPriority"

== system TurnLightLogic_backup/Runnable_sys/Function-Call Subsystem8 ==
  function : TriggerPort  TriggerType=function-call  VariantControl=(inherit)
  Bus Creator : BusCreator  Inputs=7  OutDataTypeStr=Bus: TurnLightService  NonVirtualBus=on
  Constant : Constant  Value=ComplexTurnLightOnOff.ONOFF_NOREQUEST  OutDataTypeStr=Enum: ComplexTurnLightOnOff
  Constant1 : Constant  Value=ComplexTurnLightPosition.POS_NOREQUEST  OutDataTypeStr=Enum:ComplexTurnLightPosition
  Constant2 : Constant  Value=0  OutDataTypeStr=uint8
  Constant3 : Constant  Value=8  OutDataTypeStr=uint8
  Constant4 : Constant  Value=0  OutDataTypeStr=uint8
  Constant5 : Constant  Value=0  OutDataTypeStr=uint8
  Constant6 : Constant  Value=0  VectorParams1D=off  OutDataTypeStr=uint8
  TurnLightService_TurnLightControl_Operation_Operation : FunctionCaller  FunctionPrototype=TurnLightService_TurnLightControl_Operation_Operation(TurnLightCtrlPara)  InputArgumentSpecifications=P_TurnLightService_Ctrl_Oeration
  wires:
  Constant5/1 -> Bus Creator/6  "TurnLightNum"
  Bus Creator/1 -> TurnLightService_TurnLightControl_Operation_Operation/1
  Constant/1 -> Bus Creator/2  "TurnLightOnOff"
  Constant1/1 -> Bus Creator/1  "TurnLightPosition"
  Constant3/1 -> Bus Creator/4  "TurnLightCycle"
  Constant4/1 -> Bus Creator/5  "TurnLightTimes"
  Constant2/1 -> Bus Creator/3  "TurnLightDutyCycle"
  Constant6/1 -> Bus Creator/7  "TurnLightPriority"

== system TurnLightLogic_backup/Runnable_sys/Function-Call Subsystem9 ==
  function : TriggerPort  TriggerType=function-call  VariantControl=(inherit)
  Bus Creator : BusCreator  Inputs=7  OutDataTypeStr=Bus: TurnLightService  NonVirtualBus=on
  Constant : Constant  Value=ComplexTurnLightOnOff.ON  OutDataTypeStr=Enum: ComplexTurnLightOnOff
  Constant1 : Constant  Value=ComplexTurnLightPosition.RIGHT  OutDataTypeStr=Enum:ComplexTurnLightPosition
  Constant2 : Constant  Value=0  OutDataTypeStr=uint8
  Constant3 : Constant  Value=8  OutDataTypeStr=uint8
  Constant4 : Constant  Value=0  OutDataTypeStr=uint8
  Constant5 : Constant  Value=3  OutDataTypeStr=uint8
  Constant6 : Constant  Value=3  VectorParams1D=off  OutDataTypeStr=uint8
  TurnLightService_TurnLightControl_Operation_Operation : FunctionCaller  FunctionPrototype=TurnLightService_TurnLightControl_Operation_Operation(TurnLightCtrlPara)  InputArgumentSpecifications=P_TurnLightService_Ctrl_Oeration
  wires:
  Constant6/1 -> Bus Creator/7  "TurnLightPriority"
  Constant2/1 -> Bus Creator/3  "TurnLightDutyCycle"
  Constant4/1 -> Bus Creator/5  "TurnLightTimes"
  Constant3/1 -> Bus Creator/4  "TurnLightCycle"
  Constant1/1 -> Bus Creator/1  "TurnLightPosition"
  Constant/1 -> Bus Creator/2  "TurnLightOnOff"
  Bus Creator/1 -> TurnLightService_TurnLightControl_Operation_Operation/1
  Constant5/1 -> Bus Creator/6  "TurnLightNum"

== stateflow chart TurnLightLogic_backup/Runnable_sys/HazardLogic ==
  state CrashIntensity
    en:
    HazardReq=HAZARD_ON;
  state IDLE
    en:
    HazardReq=HAZARD_OFF;
  state CheckTime
  state EmergencyBrake
    en:
    HazardReq=HAZARD_ON;
  state Hazard
    en:
    HazardReq=HAZARD_ON;
  IDLE -> IDLE [order 4] : [HazardSw_Signal==HAZARD_INACTIVE]
  (default) -> IDLE
  IDLE -> CrashIntensity [order 1] : [hasChangedFrom(CrashIntensity_Signal,HAZARD_INACTIVE)]
  CheckTime -> CheckTime [order 2] : [HazardSw_Signal==HAZARD_INACTIVE]
  CrashIntensity -> CheckTime [order 2] : [after(5,sec)]
  CheckTime -> IDLE [order 1] : [HazardSw_Signal==HAZARD_ACTIVE&&after(10,msec)]
  CrashIntensity -> IDLE [order 1] : [after(900,sec)]
  EmergencyBrake -> EmergencyBrake [order 3] : [HazardSw_Signal==HAZARD_INACTIVE]
  IDLE -> EmergencyBrake [order 2] : [hasChangedFrom(EmergencyBrakeLight_Signal,HAZARD_INACTIVE)]
  EmergencyBrake -> IDLE [order 1] : [VehicleSpeed_Signal>=15&&VehicleSpeed_Valid_Signal==ACTIVE]
  EmergencyBrake -> IDLE [order 2] : [HazardSw_Signal==HAZARD_ACTIVE&&after(10,msec)]
  Hazard -> Hazard [order 2] : [HazardSw_Signal==HAZARD_INACTIVE]
  IDLE -> Hazard [order 3] : [HazardSw_Signal==HAZARD_ACTIVE&&after(300,msec)]
  Hazard -> IDLE [order 1] : [HazardSw_Signal==HAZARD_ACTIVE&&after(300,msec)]
  data: CrashIntensity_Signal input uint8; EmergencyBrakeLight_Signal input uint8; HazardReq output uint8; HazardSw_Signal input uint8; VehicleSpeed_Signal input uint8; VehicleSpeed_Valid_Signal input uint8; ACTIVE constant uint8 =1; HAZARD_ACTIVE constant uint8 =1; HAZARD_INACTIVE constant uint8 =0; HAZARD_OFF constant uint8 =0; HAZARD_ON constant double =1; CheckTime local uint8

== stateflow chart TurnLightLogic_backup/Runnable_sys/Diagnosis ==
  state act_FL(action) [function]
    (default) -> (junction 281)
    (junction 281) -> (junction 284) [order 2]
    (junction 281) -> (junction 279) [order 1] : [token==0&&FL_flag==1]
    (junction 284) -> (junction 287)
    (junction 279) -> (junction 285) [order 2]
    (junction 285) -> (junction 280) [order 2]
    (junction 280) -> (junction 287) [order 2]
    (junction 279) -> (junction 288) [order 1] : [action==0]
    (junction 285) -> (junction 286) [order 1] : [action==1]
    (junction 280) -> (junction 290) [order 1] : [action==2]
    (junction 287) -> (junction 297)
    (junction 288) -> (junction 291) : {ClearPriority;}
    (junction 286) -> (junction 295) : {FL_OFF;}
    (junction 290) -> (junction 283) : {FL_DOUBLE;}
    (junction 291) -> (junction 295)
    (junction 295) -> (junction 283)
    (junction 283) -> (junction 297) : {FL_flag=0;}
  state Schedule
    du:
    tokenplus();
    state FL [parallel]
      settings: executionOrder=2
      state IDLE
        en:
        act_FL(0);
      state Short
        en:
        act_FL(1);
      state Long
        en:
        act_FL(2);
      (default) -> Schedule.FL.IDLE
      Schedule.FL.Short -> Schedule.FL.Short [order 2] : [FL_flag==1]
      Schedule.FL.IDLE -> Schedule.FL.IDLE [order 3] : [FL_flag==1]
      Schedule.FL.IDLE -> Schedule.FL.Short [order 1] : [TurnLampFb_FL_Signal==SHORT&&...
          | TurnLampCtrlCmd_FL_Signal==ON]{FL_flag=1;}
      Schedule.FL.Short -> Schedule.FL.IDLE [order 1] : [TurnLampFb_FL_Signal!=SHORT]{LeftRetry=1;FL_flag=1;}
      Schedule.FL.IDLE -> Schedule.FL.Long [order 2] : [TurnLampFb_FL_Signal==OPEN&&...
          | TurnLampCtrlCmd_FL_Signal==ON]{FL_flag=1;}
      Schedule.FL.Long -> Schedule.FL.IDLE [order 1] : [TurnLampFb_FL_Signal!=OPEN]{LeftRetry=1;
          | FL_flag=1;}
      Schedule.FL.Long -> Schedule.FL.Long [order 2] : [FL_flag==1]
    state RL [parallel]
      settings: executionOrder=1
      state IDLE
        en:
        act_RL(0);
      state Short
        en:
        act_RL(1);
      state Long
        en:
        act_RL(2);
      Schedule.RL.Short -> Schedule.RL.Short [order 2] : [RL_flag==1]
      (default) -> Schedule.RL.IDLE
      Schedule.RL.IDLE -> Schedule.RL.IDLE [order 3] : [RL_flag==1]
      Schedule.RL.IDLE -> Schedule.RL.Short [order 1] : [TurnLampFb_RL_Signal==SHORT&&...
          | TurnLampCtrlCmd_RL_Signal==ON]{RL_flag=1;}
      Schedule.RL.Short -> Schedule.RL.IDLE [order 1] : [TurnLampFb_RL_Signal!=SHORT]{LeftRetry=1;
          | RL_flag=1;}
      Schedule.RL.Long -> Schedule.RL.Long [order 2] : [RL_flag==1]
      Schedule.RL.IDLE -> Schedule.RL.Long [order 2] : [TurnLampFb_RL_Signal==OPEN&&...
          | TurnLampCtrlCmd_RL_Signal==ON]{RL_flag=1;}
      Schedule.RL.Long -> Schedule.RL.IDLE [order 1] : [TurnLampFb_RL_Signal!=OPEN]{LeftRetry=1;
          | RL_flag=1;}
    state FR [parallel]
      settings: executionOrder=3
      state IDLE
        en:
        act_FR(0);
      state Short
        en:
        act_FR(1);
      state Long
        en:
        act_FR(2);
      (default) -> Schedule.FR.IDLE
      Schedule.FR.IDLE -> Schedule.FR.IDLE [order 3] : [FR_flag==1]
      Schedule.FR.Short -> Schedule.FR.Short [order 2] : [FR_flag==1]
      Schedule.FR.IDLE -> Schedule.FR.Short [order 1] : [TurnLampFb_FR_Signal==SHORT&&...
          | TurnLampCtrlCmd_FR_Signal==ON]{FR_flag=1;}
      Schedule.FR.Short -> Schedule.FR.IDLE [order 1] : [TurnLampFb_FR_Signal!=SHORT]{RightRetry=1;
          | FR_flag=1;}
      Schedule.FR.Long -> Schedule.FR.Long [order 2] : [FR_flag==1]
      Schedule.FR.IDLE -> Schedule.FR.Long [order 2] : [TurnLampFb_FR_Signal==OPEN&&...
          | TurnLampCtrlCmd_FR_Signal==ON]{FR_flag=1;}
      Schedule.FR.Long -> Schedule.FR.IDLE [order 1] : [TurnLampFb_FR_Signal!=OPEN]{RightRetry=1;
          | FR_flag=1;}
    state RR [parallel]
      settings: executionOrder=4
      state IDLE
        en:
        act_RR(0);
      state Short
        en:
        act_RR(1);
      state Long
        en:
        act_RR(2);
      (default) -> Schedule.RR.IDLE
      Schedule.RR.IDLE -> Schedule.RR.IDLE [order 3] : [RR_flag==1]
      Schedule.RR.Short -> Schedule.RR.Short [order 2] : [RR_flag==1]
      Schedule.RR.IDLE -> Schedule.RR.Short [order 1] : [TurnLampFb_RR_Signal==SHORT&&...
          | TurnLampCtrlCmd_RR_Signal==ON]{RR_flag=1;}
      Schedule.RR.Short -> Schedule.RR.IDLE [order 1] : [TurnLampFb_RR_Signal!=SHORT]{RightRetry=1;
          | RR_flag=1;}
      Schedule.RR.Long -> Schedule.RR.Long [order 2] : [RR_flag==1]
      Schedule.RR.IDLE -> Schedule.RR.Long [order 2] : [TurnLampFb_RR_Signal==OPEN&&...
          | TurnLampCtrlCmd_RR_Signal==ON]{RR_flag=1;}
      Schedule.RR.Long -> Schedule.RR.IDLE [order 1] : [TurnLampFb_RR_Signal!=OPEN]{RightRetry=1;
          | RR_flag=1;}
  state tokenplus [function]
    (default) -> (junction 395)
    (junction 395) -> (junction 87) : {token++;}
    (junction 87) -> (junction 88) [order 1] : [token==4]
    (junction 88) -> (junction 90) : {token=0;}
    (junction 90) -> (junction 87)
    (junction 87) -> (junction 89) [order 2]
  state act_FR(action) [function]
    (default) -> (junction 186)
    (junction 186) -> (junction 188) [order 2]
    (junction 186) -> (junction 189) [order 1] : [token==1&&FR_flag==1]
    (junction 188) -> (junction 193)
    (junction 189) -> (junction 190) [order 2]
    (junction 190) -> (junction 181) [order 2]
    (junction 181) -> (junction 193) [order 2]
    (junction 189) -> (junction 195) [order 1] : [action==0]
    (junction 190) -> (junction 198) [order 1] : [action==1]
    (junction 181) -> (junction 199) [order 1] : [action==2]
    (junction 193) -> (junction 192)
    (junction 195) -> (junction 201) : {ClearPriority;}
    (junction 198) -> (junction 183) : {FR_OFF;}
    (junction 199) -> (junction 204) : {FR_DOUBLE;}
    (junction 201) -> (junction 183)
    (junction 183) -> (junction 204)
    (junction 204) -> (junction 192) : {FR_flag=0;}
  state act_RR(action) [function]
    (default) -> (junction 345)
    (junction 345) -> (junction 346) [order 2]
    (junction 345) -> (junction 349) [order 1] : [token==3&&RR_flag==1]
    (junction 346) -> (junction 353)
    (junction 349) -> (junction 352) [order 2]
    (junction 352) -> (junction 341) [order 2]
    (junction 341) -> (junction 353) [order 2]
    (junction 349) -> (junction 355) [order 1] : [action==0]
    (junction 352) -> (junction 347) [order 1] : [action==1]
    (junction 341) -> (junction 357) [order 1] : [action==2]
    (junction 353) -> (junction 361)
    (junction 355) -> (junction 348) : {ClearPriority;}
    (junction 347) -> (junction 359) : {RR_OFF;}
    (junction 357) -> (junction 360) : {RR_DOUBLE;}
    (junction 348) -> (junction 359)
    (junction 359) -> (junction 360)
    (junction 360) -> (junction 361) : {RR_flag=0;}
  state act_RL(action) [function]
    (default) -> (junction 313)
    (junction 313) -> (junction 316) [order 2]
    (junction 313) -> (junction 311) [order 1] : [token==2&&RL_flag==1]
    (junction 316) -> (junction 319)
    (junction 311) -> (junction 317) [order 2]
    (junction 317) -> (junction 312) [order 2]
    (junction 312) -> (junction 319) [order 2]
    (junction 311) -> (junction 320) [order 1] : [action==0]
    (junction 317) -> (junction 318) [order 1] : [action==1]
    (junction 312) -> (junction 322) [order 1] : [action==2]
    (junction 319) -> (junction 329)
    (junction 320) -> (junction 323) : {ClearPriority;}
    (junction 318) -> (junction 327) : {RL_OFF;}
    (junction 322) -> (junction 315) : {RL_DOUBLE;}
    (junction 323) -> (junction 327)
    (junction 327) -> (junction 315)
    (junction 315) -> (junction 329) : {RL_flag=0;}
  (default) -> Schedule
  data: action function_input double; action function_input double; action function_input double; action function_input double; TurnLampFb_FL_Signal input uint8; TurnLampFb_FR_Signal input uint8; TurnLampFb_RL_Signal input uint8; TurnLampFb_RR_Signal input uint8; TurnLampCtrlCmd_FL_Signal input uint8; TurnLampCtrlCmd_FR_Signal input uint8; TurnLampCtrlCmd_RL_Signal input uint8; TurnLampCtrlCmd_RR_Signal input uint8; LeftRetry data_store_memory; RightRetry data_store_memory; OPEN constant uint8 =2; ON constant uint8 =1; SHORT constant uint8 =1; token local uint8 =0; FL_flag local boolean =0; FR_flag local boolean =0; RL_flag local boolean =0; RR_flag local boolean =0
  events: FL_OFF output FUNCTION_CALL_EVENT; FL_DOUBLE output FUNCTION_CALL_EVENT; FR_DOUBLE output FUNCTION_CALL_EVENT; FR_OFF output FUNCTION_CALL_EVENT; RL_DOUBLE output FUNCTION_CALL_EVENT; RL_OFF output FUNCTION_CALL_EVENT; RR_DOUBLE output FUNCTION_CALL_EVENT; RR_OFF output FUNCTION_CALL_EVENT; ClearPriority output FUNCTION_CALL_EVENT

== stateflow chart TurnLightLogic_backup/Runnable_sys/TurnLightLogic ==
  state IDLE
    TurnLightReq=NOREQUEST;
    TurnLightMode=MODE_NOREQUEST;
  state TurnLeft
    en:
    CheckTime=0;
    TurnLightReq=TURN_LEFT;
    state Change
      du:
      CheckTime++;
    state CheckTime
      du:
      CheckTime++;
    state ShineThree
      en:
      TurnLightMode=MODE_THREE;
    state ShineLong
      en:
      TurnLightMode=MODE_LONG;
    (default) -> TurnLeft.CheckTime
    TurnLeft.CheckTime -> TurnLeft.Change : [CheckTime>=10&&...
        | TurnLampSw_Signal==TURN_LEFT]
    TurnLeft.Change -> TurnLeft.ShineThree [order 1] : [CheckTime<=80&&...
        | TurnLampSw_Signal!=TURN_LEFT]
    TurnLeft.Change -> TurnLeft.ShineLong [order 2] : [CheckTime>=80]
  state TurnRight
    en:
    CheckTime=0;
    TurnLightReq=TURN_RIGHT;
    state Change
      du:
      CheckTime++;
    state CheckTime
      du:
      CheckTime++;
    state ShineThree
      en:
      TurnLightMode=MODE_THREE;
    state ShineLong
      en:
      TurnLightMode=MODE_LONG;
    (default) -> TurnRight.CheckTime
    TurnRight.CheckTime -> TurnRight.Change : [CheckTime>=10&&...
        | TurnLampSw_Signal==TURN_RIGHT]
    TurnRight.Change -> TurnRight.ShineThree [order 1] : [CheckTime<=80&&...
        | TurnLampSw_Signal!=TURN_RIGHT]
    TurnRight.Change -> TurnRight.ShineLong [order 2] : [CheckTime>=80]
  (default) -> IDLE
  IDLE -> TurnLeft [order 1] : [(IGN_Status_Signal==IGN_ON|IGN_Status_Signal==IGNST)&&...
      | TurnLampSw_Signal==TURN_LEFT]
  TurnLeft -> IDLE : [IGN_Status_Signal==IGN_OFF]
  TurnLeft.ShineThree -> IDLE : [CountSignal_Left_Signal==3]
  TurnLeft.ShineLong -> IDLE : [TurnLampSw_Signal!=TURN_LEFT]
  IDLE -> TurnRight [order 2] : [(IGN_Status_Signal==IGN_ON|IGN_Status_Signal==IGNST)&&...
      | TurnLampSw_Signal==TURN_RIGHT]
  TurnRight -> IDLE : [IGN_Status_Signal==IGN_OFF]
  TurnRight.ShineThree -> IDLE : [CountSignal_Right_Signal==3]
  TurnRight.ShineLong -> IDLE : [TurnLampSw_Signal!=TURN_RIGHT]
  data: CountSignal_Left_Signal input uint8; CountSignal_Right_Signal input uint8; IGN_Status_Signal input uint8; TurnLampSw_Signal input uint8; TurnLightReq output uint8; TurnLightMode output uint8; CheckTime local uint16; IGNST constant uint8 =3; IGN_OFF constant uint8 =0; IGN_ON constant uint8 =1; MODE_LONG constant uint8 =2; MODE_NOREQUEST constant uint8 =0; MODE_THREE constant uint8 =1; NOREQUEST constant uint8 =0; TURN_LEFT constant uint8 =1; TURN_RIGHT constant uint8 =2

== stateflow chart TurnLightLogic_backup/Runnable_sys/TurnLightSelector ==
  state ALLOFF
    en:
    TurnLight_ALLOFF
  state delay2
  state Left_ON
    en:
    LeftShortOrLong();
    LeftRetry=0;
  state LeftShortOrLong [function]
    (default) -> (junction 30)
    (junction 30) -> (junction 31) [order 1] : [TurnLightMode==MODE_THREE]
    (junction 30) -> (junction 32) [order 2] : {TurnLight_LeftLong;}
    (junction 31) -> (junction 33) : {TurnLight_LeftShort;}
    (junction 33) -> (junction 32)
    (junction 32) -> (junction 34)
  state delay1
  state Right_ON
    en:
    RightShortOrLong();
    RightRetry=0;
  state RightShortOrLong [function]
    (default) -> (junction 37)
    (junction 37) -> (junction 36) [order 1] : [TurnLightMode==MODE_THREE]
    (junction 37) -> (junction 40) [order 2] : {TurnLight_RightLong;}
    (junction 36) -> (junction 41) : {TurnLight_RightShort;}
    (junction 41) -> (junction 40)
    (junction 40) -> (junction 38)
  state delay
  state Hazard_ON
    en:
    TurnLight_ALLON;
    LeftRetry=0;
    RightRetry=0;
  (default) -> ALLOFF
  delay2 -> Left_ON : [after(500,msec)]
  Left_ON -> delay2 [order 2] : [LeftRetry==1]
  ALLOFF -> Left_ON [order 1] : [TurnLightReq==TURN_LEFT]
  Left_ON -> (junction 47) [order 3] : [HazardReq==HAZARD_ON&&...
      | hasChangedFrom(TurnLightReq,TURN_LEFT)]
  (junction 47) -> (junction 48)
  Left_ON -> (junction 52) [order 4] : [TurnLightReq==TURN_LEFT&&...
      | hasChangedTo(HazardReq,HAZARD_ON)]
  (junction 52) -> (junction 53)
  Left_ON -> ALLOFF [order 1] : [TurnLightReq!=TURN_LEFT]
  (junction 92) -> Left_ON : [TurnLightReq==TURN_LEFT&&...
      | hasChangedTo(HazardReq,HAZARD_OFF)]
  (junction 90) -> (junction 92)
  delay1 -> Right_ON : [after(500,msec)]
  Right_ON -> delay1 [order 2] : [RightRetry==1]
  ALLOFF -> Right_ON [order 2] : [TurnLightReq==TURN_RIGHT]
  (junction 84) -> Right_ON : [TurnLightReq==TURN_RIGHT&&...
      | hasChangedTo(HazardReq,HAZARD_OFF)]
  (junction 82) -> (junction 84)
  Right_ON -> (junction 69) [order 3] : [HazardReq==HAZARD_ON&&...
      | hasChangedFrom(TurnLightReq,TURN_RIGHT)]
  (junction 69) -> (junction 74)
  Right_ON -> (junction 67) [order 4] : [TurnLightReq==TURN_RIGHT&&...
      | hasChangedTo(HazardReq,HAZARD_ON)]
  Right_ON -> ALLOFF [order 1] : [TurnLightReq!=TURN_RIGHT]
  (junction 67) -> (junction 76)
  delay -> Hazard_ON : [after(500,msec)]
  Hazard_ON -> delay [order 4] : [LeftRetry==1||RightRetry==1]
  (junction 76) -> Hazard_ON
  (junction 74) -> Hazard_ON
  ALLOFF -> Hazard_ON [order 3] : [HazardReq==HAZARD_ON]
  Hazard_ON -> (junction 82) [order 3]
  Hazard_ON -> (junction 90) [order 1]
  (junction 53) -> Hazard_ON
  Hazard_ON -> ALLOFF [order 2] : [HazardReq==HAZARD_OFF]
  (junction 48) -> Hazard_ON
  data: TurnLightReq input uint8; TurnLightMode input uint8; HazardReq input uint8; LeftRetry data_store_memory; RightRetry data_store_memory; HAZARD_OFF constant uint8 =0; HAZARD_ON constant uint8 =1; MODE_THREE constant uint8 =1; TURN_LEFT constant uint8 =1; TURN_RIGHT constant uint8 =2
  events: TurnLight_RightShort output FUNCTION_CALL_EVENT; TurnLight_RightLong output FUNCTION_CALL_EVENT; TurnLight_LeftShort output FUNCTION_CALL_EVENT; TurnLight_LeftLong output FUNCTION_CALL_EVENT; TurnLight_ALLON output FUNCTION_CALL_EVENT; TurnLight_ALLOFF output FUNCTION_CALL_EVENT
